simulink subsystem "Magnetometer"  (R2023a)
settings: Solver=VariableStepAuto  StartTime=0.0  StopTime=10.0  RelTol=1e-3
undefined symbols (not defined in the file or in its folder): WMM2020
libraries: aerolibgravity2 x1
settings Model: Creator=jonvargas  LastModifiedBy=jonvargas

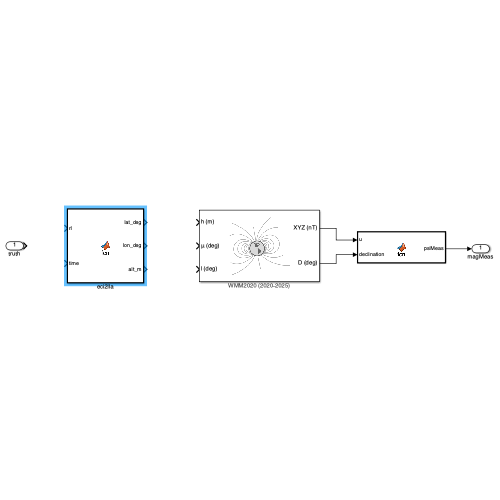
[thumbnail: Simulink's stored preview of the top-level diagram]
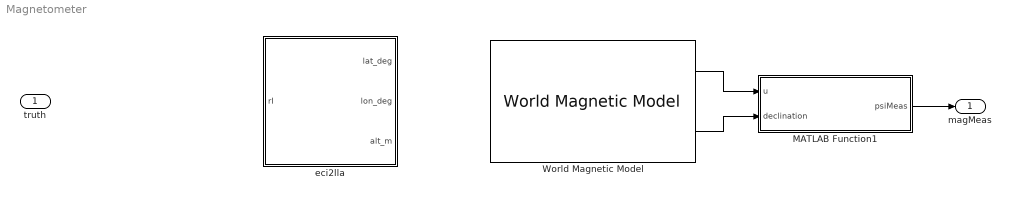
== system Magnetometer ==
  truth : Inport
  MATLAB Function1 : MATLAB Function  TreatAsAtomicUnit=on
  World Magnetic Model : aerolibgravity2/World Magnetic Model  model=WMM2020 (2020-2025)  customFile='WMM2020.COF'  units=Metric (MKS)  time_in=off  month=January  day=1  year=2025  action=Error  h_out=off  dec_out=on  inc_out=off  ti_out=off
  eci2lla : MATLAB Function  TreatAsAtomicUnit=on
  magMeas : Outport
  wires:
  World Magnetic Model/1 -> MATLAB Function1/1(u)
  World Magnetic Model/2 -> MATLAB Function1/2(declination)
  MATLAB Function1/1(psiMeas) -> magMeas/1

== matlab function Magnetometer/MATLAB Function1 ==
  data: u input; psiMeas output; declination input
function psiMeas = fcn(u, declination)

psi = atan(u(2),u(3));
psiMeas = psi - declination;

== matlab function Magnetometer/eci2lla ==
  data: lat_deg output; rI input; params parameter; lon_deg output; alt_m output
function [lat_deg,lon_deg,alt_m] = fcn(rI,params)

% Inertial to ECEF rotation
Ci2e = Reci2ecef(params,time);
rE_m = Ci2e*rI_m;

[LLA] = ecef2geodetic(rE_m);
lat_deg = LLA(1,:);
lon_deg = LLA(2,:);
alt_m = LLA(3,:);
